simulink model "hdl_model_fixed"  (R2024a)
settings: Solver=VariableStepAuto  StartTime=0.0  StopTime=2  RelTol=1e-3
values from neighbouring files (symbols this model uses):
  BUFFER_LEN = 2048    [workspace.mat]
  SAMPLING_FREQ = 12800    [workspace.mat]
  signal_1 = [0 0.0001 0.0002 0.0003 0.0004 0.0005 0.0006 0.0007 0.0008 0.0009 0.001 0.0011 ... (4096 elements, 2048x2)]    [workspace.mat]
libraries: hdlsllib x2, dspsrcs4 x1, dsphdlxfrm2 x1, simulink_extras x1, dspsigops x1, simulink x1
settings Model: SimulationMode=accelerator  Creator=Jan Rosa  LastModifiedBy=Jan Rosa
settings DebuggingCC: SignalRangeChecking=warning

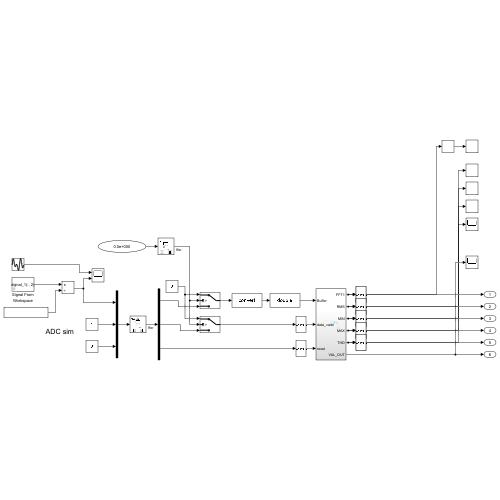
[thumbnail: Simulink's stored preview of the top-level diagram]
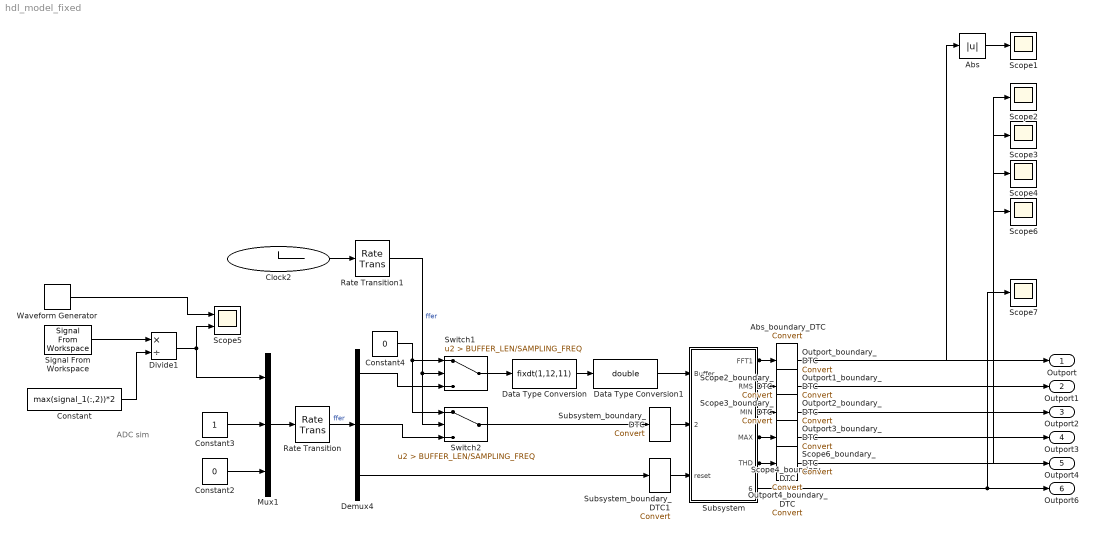
== system hdl_model_fixed ==
  note: ADC sim
  Abs : Abs  SaturateOnIntegerOverflow=off
  Abs_boundary_DTC : DataTypeConversion
  Clock2 : Clock
  Constant : Constant  Value=max(signal_1(:,2))*2
  Constant2 : Constant  Value=0
  Constant3 : Constant
  Constant4 : Constant  Value=0  SampleTime=1/SAMPLING_FREQ
  Data Type Conversion : DataTypeConversion  OutDataTypeStr=fixdt(1,12,11)  SaturateOnIntegerOverflow=off  RndMeth=Floor
  Data Type Conversion1 : DataTypeConversion  OutDataTypeStr=double  SaturateOnIntegerOverflow=off  RndMeth=Floor
  Demux4 : Demux  Outputs=3
  Divide1 : Product  Inputs=*/
  Mux1 : Mux  Inputs=3
  Outport1_boundary_DTC : DataTypeConversion
  Outport2_boundary_DTC : DataTypeConversion
  Outport3_boundary_DTC : DataTypeConversion
  Outport4_boundary_DTC : DataTypeConversion
  Outport_boundary_DTC : DataTypeConversion
  Rate Transition : RateTransition  Integrity=off  Deterministic=off  OutPortSampleTime=1/SAMPLING_FREQ
  Rate Transition1 : RateTransition  Integrity=off  Deterministic=off  OutPortSampleTime=1/SAMPLING_FREQ
  Scope{1..4,6..7} (6 alike) : Scope
  Scope2_boundary_DTC : DataTypeConversion
  Scope3_boundary_DTC : DataTypeConversion
  Scope4_boundary_DTC : DataTypeConversion
  Scope5 : Scope  NumInputPorts=2
  Scope6_boundary_DTC : DataTypeConversion
  Signal From Workspace : dspsrcs4/Signal From Workspace  X=signal_1(:, 2)  Ts=signal_1(2, 1)  nsamps=1  OutputAfterFinalValue=Cyclic repetition  ignoreOrWarnInputAndFrameLengths=off  OutputFrames=off
  Subsystem : Subsystem
  Subsystem_boundary_DTC : DataTypeConversion
  Subsystem_boundary_DTC1 : DataTypeConversion
  Switch1 : Switch  Criteria=u2 > Threshold  Threshold=BUFFER_LEN/SAMPLING_FREQ  SaturateOnIntegerOverflow=off  InputSameDT=off
  Switch2 : Switch  Criteria=u2 > Threshold  Threshold=BUFFER_LEN/SAMPLING_FREQ  SaturateOnIntegerOverflow=off  InputSameDT=off
  Waveform Generator : simulink/Sources/Waveform Generator  OutMin=[]  OutMax=[]  OutDataTypeStr=double  SelectedSignal=1  Signals=0.99*sin(0.5, 50*2*pi, 0)  BlockNames=MultiportSwitch_c7ceefe4d1e8441  SampleTime=1/(SAMPLING_FREQ*2)
  Outport : Outport
  Outport1 : Outport  Port=2
  Outport2 : Outport  Port=3
  Outport3 : Outport  Port=4
  Outport4 : Outport  Port=5
  Outport6 : Outport  Port=6
  wires:
  Constant3/1 -> Mux1/2
  Subsystem/3(MIN) -> Scope3_boundary_DTC/1, Outport2_boundary_DTC/1
  Rate Transition1/1 -> Switch2/2, Switch1/2  "ffer"
  Rate Transition/1 -> Demux4/1  "ffer"
  Constant4/1 -> Switch2/1, Switch1/1
  Constant/1 -> Divide1/2
  Clock2/1 -> Rate Transition1/1
  Subsystem/1(FFT1) -> Abs_boundary_DTC/1, Outport_boundary_DTC/1
  Subsystem/6(VAL_OUT) -> Outport6/1, Scope7/1
  Mux1/1 -> Rate Transition/1
  Demux4/1 -> Switch1/3
  Signal From Workspace/1 -> Divide1/1
  Switch1/1 -> Data Type Conversion/1
  Abs/1 -> Scope1/1
  Divide1/1 -> Mux1/1, Scope5/2
  Subsystem/5(THD) -> Scope6_boundary_DTC/1, Outport4_boundary_DTC/1
  Demux4/2 -> Switch2/3
  Subsystem/4(MAX) -> Scope4_boundary_DTC/1, Outport3_boundary_DTC/1
  Subsystem/2(RMS) -> Scope2_boundary_DTC/1, Outport1_boundary_DTC/1
  Waveform Generator/1 -> Scope5/1
  Constant2/1 -> Mux1/3
  Data Type Conversion/1 -> Data Type Conversion1/1
  Data Type Conversion1/1 -> Subsystem/1(Buffer)
  Switch2/1 -> Subsystem_boundary_DTC/1
  Subsystem_boundary_DTC/1 -> Subsystem/2(data_valid)
  Demux4/3 -> Subsystem_boundary_DTC1/1
  Subsystem_boundary_DTC1/1 -> Subsystem/3(reset)
  Abs_boundary_DTC/1 -> Abs/1
  Outport_boundary_DTC/1 -> Outport/1
  Scope2_boundary_DTC/1 -> Scope2/1
  Outport1_boundary_DTC/1 -> Outport1/1
  Scope3_boundary_DTC/1 -> Scope3/1
  Outport2_boundary_DTC/1 -> Outport2/1
  Scope4_boundary_DTC/1 -> Scope4/1
  Outport3_boundary_DTC/1 -> Outport3/1
  Scope6_boundary_DTC/1 -> Scope6/1
  Outport4_boundary_DTC/1 -> Outport4/1

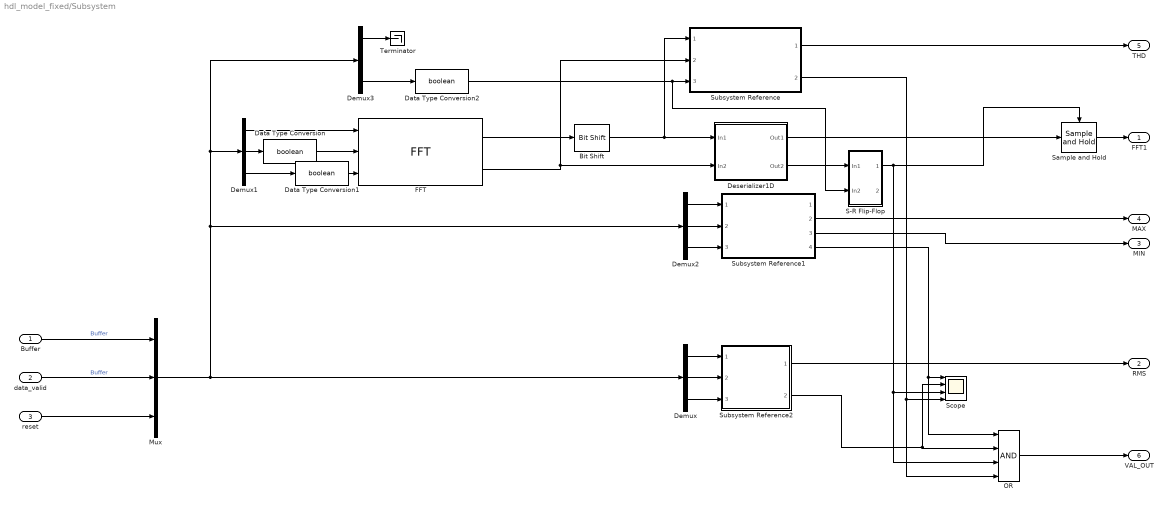
== system hdl_model_fixed/Subsystem ==
  Buffer : Inport
  data_valid : Inport  Port=2
  reset : Inport  Port=3
  Bit Shift : hdlsllib/Logic and Bit Operations/Bit Shift  mode=Shift Right Arithmetic  N=log2(BUFFER_LEN)
  Data Type Conversion : DataTypeConversion  OutDataTypeStr=boolean  SaturateOnIntegerOverflow=off  RndMeth=Floor
  Data Type Conversion1 : DataTypeConversion  OutDataTypeStr=boolean  SaturateOnIntegerOverflow=off  RndMeth=Floor
  Data Type Conversion2 : DataTypeConversion  OutDataTypeStr=boolean  SaturateOnIntegerOverflow=off  RndMeth=Floor
  Demux{,1..3} (4 alike) : Demux  Outputs=3
  Deserializer1D : Subsystem  Tag=DecoupledSystem
  FFT : dsphdlxfrm2/FFT  Architecture=Streaming Radix 2^2  FFTLengthSource=Property  FFTLength=BUFFER_LEN  FFTLengthMax=1024  ComplexMultiplication=Use 4 multipliers and 2 adders  BitReversedOutput=off  BitReversedInput=off  Normalize=off  SimulateUsing=Code generation  RoundingMethod=Floor  ResetInputPort=on  StartOutputPort=off  EndOutputPort=off
  Mux : Mux  Inputs=3
  OR : Logic  Inputs=4  IconShape=distinctive  AllPortsSameDT=off  OutDataTypeStr=boolean
  S-R Flip-Flop : Subsystem  Tag=DecoupledSystem
  Sample and Hold : dspsigops/Sample and Hold  trig=Rising edge  initCond=0  latchinput=off
  Scope : Scope  NumInputPorts=4
  Subsystem Reference : Subsystem  ReferencedSubsystem=myTHD_fixed
  Subsystem Reference1 : Subsystem  ReferencedSubsystem=BUF_MIN_MAX_AVG_fixed
  Subsystem Reference2 : Subsystem  ReferencedSubsystem=myRMS_fixed
  Terminator : Terminator
  FFT1 : Outport
  RMS : Outport  Port=2
  MIN : Outport  Port=3
  MAX : Outport  Port=4
  THD : Outport  Port=5
  VAL_OUT : Outport  Port=6
  wires:
  Subsystem Reference/1 -> THD/1
  Demux/2 -> Subsystem Reference2/2
  Demux2/2 -> Subsystem Reference1/2
  S-R Flip-Flop/1(Out1) -> Scope/3, OR/3, Sample and Hold/Trigger
  Demux2/3 -> Subsystem Reference1/3
  Subsystem Reference1/3 -> MIN/1
  Subsystem Reference1/2 -> MAX/1
  Subsystem Reference1/4 -> OR/1, Scope/1
  Demux1/3 -> Data Type Conversion1/1
  reset/1 -> Mux/3
  Demux/1 -> Subsystem Reference2/1
  Data Type Conversion/1 -> FFT/2
  OR/1 -> VAL_OUT/1
  Subsystem Reference2/2 -> OR/2, Scope/2
  Mux/1 -> Demux2/1, Demux3/1, Demux1/1, Demux/1
  Data Type Conversion1/1 -> FFT/3
  Demux/3 -> Subsystem Reference2/3
  Demux1/1 -> FFT/1
  FFT/2 -> Subsystem Reference/2, Deserializer1D/2(In2)
  Demux1/2 -> Data Type Conversion/1
  Buffer/1 -> Mux/1  "Buffer"
  data_valid/1 -> Mux/2  "Buffer"
  Subsystem Reference/2 -> OR/4, Scope/4
  Bit Shift/1 -> Subsystem Reference/1, Deserializer1D/1(In1)
  FFT/1 -> Bit Shift/1
  Deserializer1D/2(Out2) -> S-R Flip-Flop/1(In1)
  Subsystem Reference2/1 -> RMS/1
  Demux3/3 -> Data Type Conversion2/1
  Deserializer1D/1(Out1) -> Sample and Hold/1
  Sample and Hold/1 -> FFT1/1
  Data Type Conversion2/1 -> Subsystem Reference/3, S-R Flip-Flop/2(In2)
  Demux2/1 -> Subsystem Reference1/1
  Demux3/1 -> Terminator/1

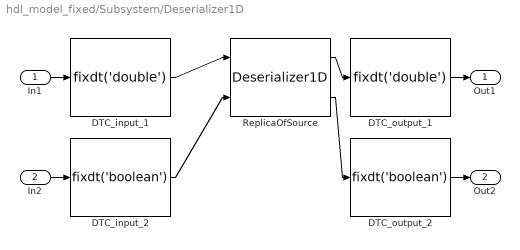
== system hdl_model_fixed/Subsystem/Deserializer1D ==
  In1 : Inport  LockScale=on
  In2 : Inport  Port=2  LockScale=on
  DTC_input_1 : DataTypeConversion  OutDataTypeStr=fixdt('double')  RndMeth=Nearest  SaturateOnIntegerOverflow=off  LockScale=on
  DTC_input_2 : DataTypeConversion  OutDataTypeStr=fixdt('boolean')  RndMeth=Nearest  SaturateOnIntegerOverflow=off  LockScale=on
  DTC_output_1 : DataTypeConversion  OutDataTypeStr=fixdt('double')  SaturateOnIntegerOverflow=off  RndMeth=Floor
  DTC_output_2 : DataTypeConversion  OutDataTypeStr=fixdt('boolean')  SaturateOnIntegerOverflow=off  RndMeth=Floor
  ReplicaOfSource : hdlsllib/HDL Operations/Deserializer1D  Ratio=BUFFER_LEN  IdleCycles=0  InitialCondition=0  startIn=off  validIn=on  validOut=on  inputDataDimensions=-1  inputSampleTime=-1  inputSignalType=auto
  Out1 : Outport  LockScale=on
  Out2 : Outport  Port=2  LockScale=on
  wires:
  DTC_output_1/1 -> Out1/1
  In2/1 -> DTC_input_2/1
  DTC_output_2/1 -> Out2/1
  In1/1 -> DTC_input_1/1
  ReplicaOfSource/1 -> DTC_output_1/1
  DTC_input_1/1 -> ReplicaOfSource/1
  ReplicaOfSource/2 -> DTC_output_2/1
  DTC_input_2/1 -> ReplicaOfSource/2

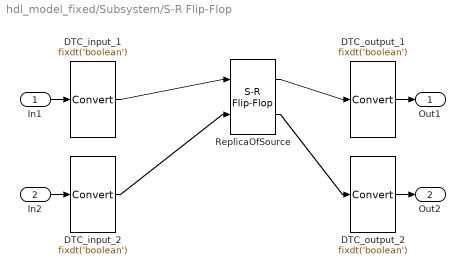
== system hdl_model_fixed/Subsystem/S-R Flip-Flop ==
  In1 : Inport  LockScale=on
  In2 : Inport  Port=2  LockScale=on
  DTC_input_1 : DataTypeConversion  OutDataTypeStr=fixdt('boolean')  RndMeth=Nearest  SaturateOnIntegerOverflow=off  LockScale=on
  DTC_input_2 : DataTypeConversion  OutDataTypeStr=fixdt('boolean')  RndMeth=Nearest  SaturateOnIntegerOverflow=off  LockScale=on
  DTC_output_1 : DataTypeConversion  OutDataTypeStr=fixdt('boolean')  SaturateOnIntegerOverflow=off  RndMeth=Floor
  DTC_output_2 : DataTypeConversion  OutDataTypeStr=fixdt('boolean')  SaturateOnIntegerOverflow=off  RndMeth=Floor
  ReplicaOfSource : simulink_extras/Flip Flops/S-R Flip-Flop  initial_condition=0
  Out1 : Outport  LockScale=on
  Out2 : Outport  Port=2  LockScale=on
  wires:
  In1/1 -> DTC_input_1/1
  DTC_input_2/1 -> ReplicaOfSource/2
  ReplicaOfSource/2 -> DTC_output_2/1
  DTC_output_1/1 -> Out1/1
  ReplicaOfSource/1 -> DTC_output_1/1
  In2/1 -> DTC_input_2/1
  DTC_input_1/1 -> ReplicaOfSource/1
  DTC_output_2/1 -> Out2/1
